simulink model "DC_charging_reqs_8_5_6_4"  (R2024b)
settings: Solver=VariableStepAuto  StartTime=0.0  StopTime=10.0  RelTol=1e-3
libraries: raptor_j1939_lib x2
settings Model: Creator=malul  LastModifiedBy=malul

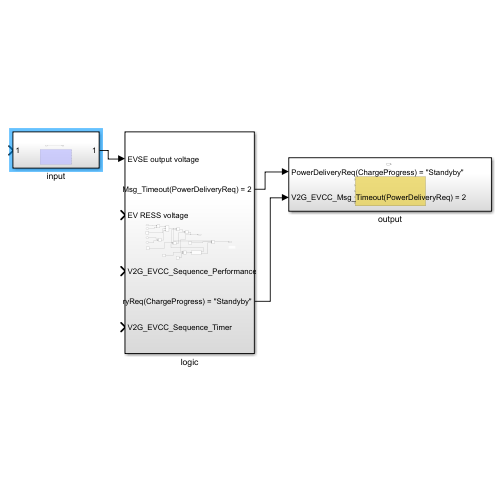
[thumbnail: Simulink's stored preview of the top-level diagram]
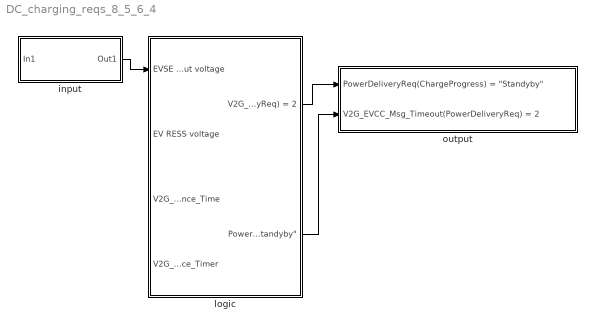
== system DC_charging_reqs_8_5_6_4 ==
  input : Subsystem
  logic : Subsystem
  output : Subsystem
  wires:
  input/1(Out1) -> logic/1(EVSE output voltage)
  logic/1(V2G_EVCC_Msg_Timeout(PowerDeliveryReq) = 2) -> output/1("PowerDeliveryReq(ChargeProgress) = \"Standyby\"")
  logic/2("PowerDeliveryReq(ChargeProgress) = \"Standyby\"") -> output/2(V2G_EVCC_Msg_Timeout(PowerDeliveryReq) = 2)

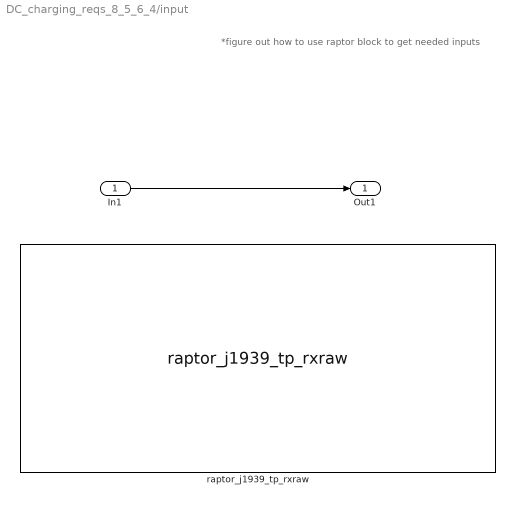
== system DC_charging_reqs_8_5_6_4/input ==
  note: *figure out how to use raptor block to get needed inputs
  In1 : Inport
  raptor_j1939_tp_rxraw : raptor_j1939_lib/Transport Protocol/raptor_j1939_tp_rxraw  bus='J1939_1'  pgn=0
      settings: SourceProductName=Raptor-J1939
  Out1 : Outport
  wires:
  In1/1 -> Out1/1

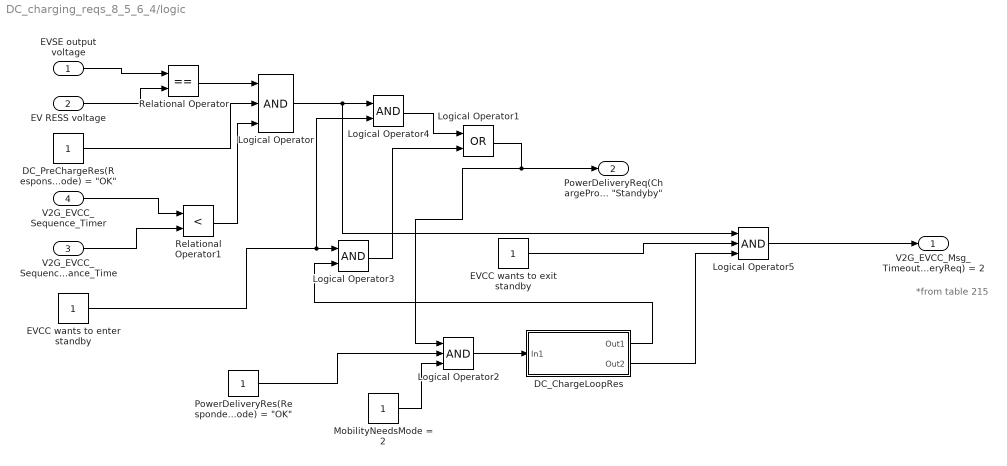
== system DC_charging_reqs_8_5_6_4/logic ==
  note: *from table 215
  EVSE output voltage : Inport
  EV RESS voltage : Inport  Port=2
  V2G_EVCC_Sequence_Performance_Time : Inport  Port=3
  V2G_EVCC_Sequence_Timer : Inport  Port=4
  DC_ChargeLoopRes : Subsystem
  "DC_PreChargeRes(ResponseCode) = \"OK\"" : Constant
  EVCC wants to enter standby : Constant
  EVCC wants to exit standby : Constant
  Logical Operator : Logic  Inputs=3  AllPortsSameDT=off  OutDataTypeStr=boolean
  Logical Operator1 : Logic  Operator=OR  AllPortsSameDT=off  OutDataTypeStr=boolean
  Logical Operator2 : Logic  Inputs=3  AllPortsSameDT=off  OutDataTypeStr=boolean
  Logical Operator3 : Logic  AllPortsSameDT=off  OutDataTypeStr=boolean
  Logical Operator4 : Logic  AllPortsSameDT=off  OutDataTypeStr=boolean
  Logical Operator5 : Logic  Inputs=3  AllPortsSameDT=off  OutDataTypeStr=boolean
  MobilityNeedsMode = 2 : Constant
  "PowerDeliveryRes(RespondeCode) = \"OK\"" : Constant
  Relational Operator : RelationalOperator  Operator===  OutDataTypeStr=boolean  RndMeth=Simplest  InputSameDT=off
  Relational Operator1 : RelationalOperator  Operator=<  OutDataTypeStr=boolean  RndMeth=Simplest  InputSameDT=off
  V2G_EVCC_Msg_Timeout(PowerDeliveryReq) = 2 : Outport
  "PowerDeliveryReq(ChargeProgress) = \"Standyby\"" : Outport  Port=2
  wires:
  EVSE output voltage/1 -> Relational Operator/1
  EV RESS voltage/1 -> Relational Operator/2
  Relational Operator/1 -> Logical Operator/1
  "DC_PreChargeRes(ResponseCode) = \"OK\""/1 -> Logical Operator/2
  V2G_EVCC_Sequence_Timer/1 -> Relational Operator1/1
  V2G_EVCC_Sequence_Performance_Time/1 -> Relational Operator1/2
  Relational Operator1/1 -> Logical Operator/3
  Logical Operator1/1 -> Logical Operator2/1, "PowerDeliveryReq(ChargeProgress) = \"Standyby\""/1
  Logical Operator/1 -> Logical Operator5/1, Logical Operator4/1
  "PowerDeliveryRes(RespondeCode) = \"OK\""/1 -> Logical Operator2/2
  MobilityNeedsMode = 2/1 -> Logical Operator2/3
  EVCC wants to enter standby/1 -> Logical Operator4/2, Logical Operator3/1
  Logical Operator2/1 -> DC_ChargeLoopRes/1(In1)
  DC_ChargeLoopRes/1(Out1) -> Logical Operator3/2
  Logical Operator3/1 -> Logical Operator1/2
  Logical Operator4/1 -> Logical Operator1/1
  EVCC wants to exit standby/1 -> Logical Operator5/2
  DC_ChargeLoopRes/2(Out2) -> Logical Operator5/3
  Logical Operator5/1 -> V2G_EVCC_Msg_Timeout(PowerDeliveryReq) = 2/1

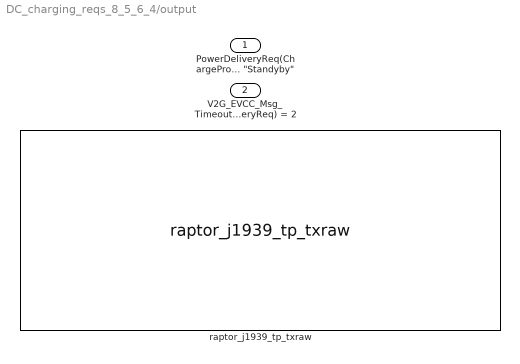
== system DC_charging_reqs_8_5_6_4/output ==
  "PowerDeliveryReq(ChargeProgress) = \"Standyby\"" : Inport
  V2G_EVCC_Msg_Timeout(PowerDeliveryReq) = 2 : Inport  Port=2
  raptor_j1939_tp_txraw : raptor_j1939_lib/Transport Protocol/raptor_j1939_tp_txraw  bus='J1939_1'  pgnNum=65207  txMode=On Request Only  period=100
      settings: SourceProductName=Raptor-J1939

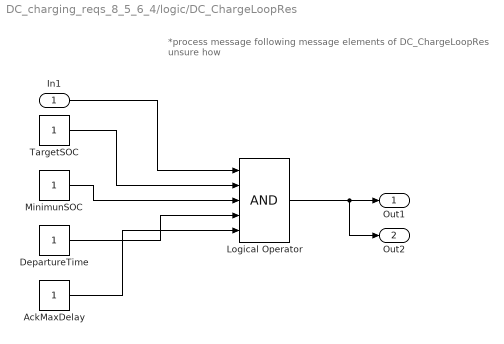
== system DC_charging_reqs_8_5_6_4/logic/DC_ChargeLoopRes ==
  note: *process message following message elements of DC_ChargeLoopRes
      |  unsure how
  In1 : Inport
  AckMaxDelay : Constant
  DepartureTime : Constant
  Logical Operator : Logic  Inputs=5  AllPortsSameDT=off  OutDataTypeStr=boolean
  MinimunSOC : Constant
  TargetSOC : Constant
  Out1 : Outport
  Out2 : Outport  Port=2
  wires:
  In1/1 -> Logical Operator/1
  TargetSOC/1 -> Logical Operator/2
  MinimunSOC/1 -> Logical Operator/3
  DepartureTime/1 -> Logical Operator/4
  AckMaxDelay/1 -> Logical Operator/5
  Logical Operator/1 -> Out2/1, Out1/1
